simulink model "sys_zn1"  (R2023b)
settings: Solver=ode8  StartTime=0.0  StopTime=t_end  FixedStep=0.01  RelTol=1e-3
values from neighbouring files (symbols this model uses):
  Kd = 1    [sim_zn1.m]
  Ki = 0.3    [sim_zn1.m]
  Kp = 0.4    [sim_zn1.m]
settings Model: Creator=suvo  LastModifiedBy=suvo
settings DataIOCC: ReturnWorkspaceOutputs=off

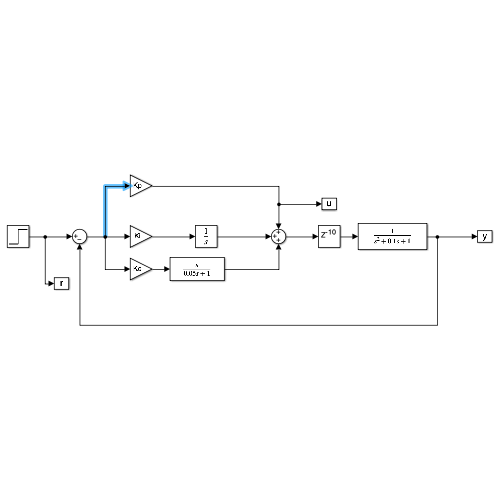
[thumbnail: Simulink's stored preview of the top-level diagram]
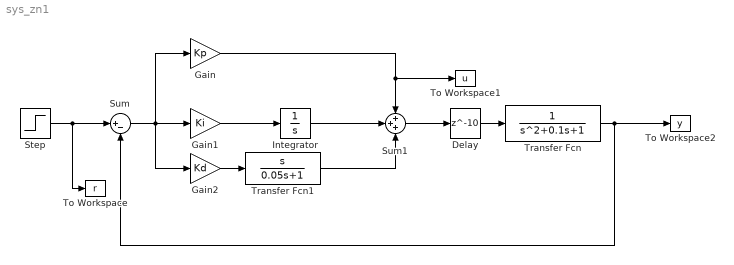
== system sys_zn1 ==
  Delay : Delay  DelayLength=10
  Gain : Gain  Gain=Kp
  Gain1 : Gain  Gain=Ki
  Gain2 : Gain  Gain=Kd
  Integrator : Integrator
  Step : Step  SampleTime=0
  Sum : Sum  Inputs=|+-
  Sum1 : Sum  Inputs=+++
  To Workspace : ToWorkspace  VariableName=r  SaveFormat=Timeseries  SampleTime=-1
  To Workspace1 : ToWorkspace  VariableName=u  SaveFormat=Timeseries  SampleTime=-1
  To Workspace2 : ToWorkspace  VariableName=y  SaveFormat=Timeseries  SampleTime=-1
  Transfer Fcn : TransferFcn  Numerator=1  Denominator=[1 0.1 1]
  Transfer Fcn1 : TransferFcn  Numerator=[1 0]  Denominator=[0.05 1]
  wires:
  Gain/1 -> To Workspace1/1, Sum1/1
  Sum/1 -> Gain2/1, Gain1/1, Gain/1
  Step/1 -> To Workspace/1, Sum/1
  Transfer Fcn/1 -> To Workspace2/1, Sum/2
  Delay/1 -> Transfer Fcn/1
  Gain1/1 -> Integrator/1
  Integrator/1 -> Sum1/2
  Gain2/1 -> Transfer Fcn1/1
  Transfer Fcn1/1 -> Sum1/3
  Sum1/1 -> Delay/1
